simulink model "tremolovariaciondevolumen"  (R2020a)
settings: Solver=VariableStepAuto  StartTime=0.0  StopTime=10  RelTol=1e-3
libraries: dspsnks4 x1, dspvision x1, dspsrcs4 x1
settings Model: Creator=TATTO PC  LastModifiedBy=TATTO PC

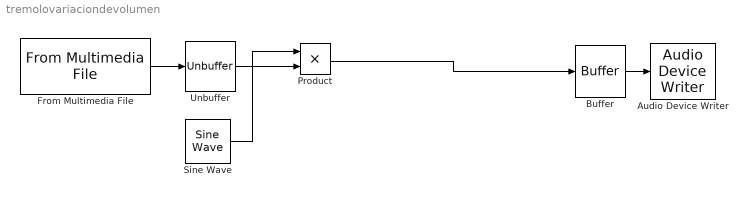
== system tremolovariaciondevolumen ==
  Audio Device Writer : dspsnks4/Audio Device Writer  Driver=DirectSound  Device=Default  InheritSampleRate=on  SampleRate=44100  BitDepth=16-bit integer  BufferSize=4096  NumBuffers=10  DefaultOutputChannelMapping=on  OutputChannelMapping=1:2  OutputNumUnderrunSamples=off  DriverIdx=1  DeviceWarnFlag=''
  Buffer : Buffer  OutputFrames=off
  From Multimedia File : dspvision/From Multimedia File  inputFilename=A:\Usuarios\TATTO PC\Desktop\univesidad\Procesamiento video y audio\Gravar un sonido clase 4\son1.wav  readRange=[1 Inf]  loop=on  numPlays=inf  outputStreams=Audio only  videoDataType=single  audioDataType=double  inheritSampleTime=on  userDefinedSampleTime=1/30  noAudioOutput=off  isIntensityVideo=off  fourcc=RGB  colorVideoFormat=Separate color signals  outputEOF=off  dataOrg=Column-major  audioFrameSize=1024  computeAudioFrameSize=off  outSamplingMode=Sample based
  Product : Product
  Sine Wave : dspsrcs4/Sine Wave  Amplitude=1  Frequency=0.2  Phase=0  SampleMode=Discrete  OutComplex=Real  CompMethod=Trigonometric fcn  TableSize=Speed  SampleTime=0.01  SamplesPerFrame=1  ResetState=Restart at time zero  OutputFrames=off  dataType=double  wordLen=16  udDataType=sfix(16)  fracBitsMode=Best precision  numFracBits=15  OutDataTypeStr=double  LastOutDataTypeStr=double
  Unbuffer : Unbuffer
  wires:
  From Multimedia File/1 -> Unbuffer/1
  Buffer/1 -> Audio Device Writer/1
  Product/1 -> Buffer/1
  Unbuffer/1 -> Product/2
  Sine Wave/1 -> Product/1
